simulink model "FinSimLagrange1"  (R2020b)
settings: Solver=FixedStepAuto  StartTime=0.0  StopTime=10.0  FixedStep=0.001  RelTol=1e-3
values from neighbouring files (symbols this model uses):
  m = {0 0 0 0 0}    [DynMatrixCalculator.m]    (also in DynMats_Iterative.mat = ; FinLagrange_2.m = mass{i})
  N = {zeros(3,1) zeros(3,1) zeros(3,1) zeros(3,1) zeros(3,1)}    [DynMatrixCalculator.m]    (also in DynMats_Iterative.mat = )
undefined symbols (not defined in the file or in its folder): X, Y, Z
libraries: sm_lib x34, nesl_utility x24
(part 4 of 4)

== matlab function FinSimLagrange1/Analytical Forward. Dynamics/MATLAB Function ==
  data: Tau input; theta input; theta_d input; theta_2d output; EndEffector output
function [theta_2d,EndEffector] = fcn(Tau, theta, theta_d)

q1 = theta(1);    q_d1 = theta_d(1);
q2 = theta(2);    q_d2 = theta_d(2);
q3 = theta(3);    q_d3 = theta_d(3);
q4 = theta(4);    q_d4 = theta_d(4);

%% M
M= [                                                                                                                                                                                                                                                                                                                                                                                                                                            27947/500,                                                                                                                                                                                                                                                                                                                                                                                                                                                                                                                                                                                                                                                                                                                                                                                                                                                                                                                                                                                                                                                                                                                                                                                                                                                                                                                                                                                                                                                                                                                                                                                                                                                                                                                                                                                                                                                                                                                                                                                                                                                                                                                                                                                                                                                                                                                                                                                                                                                                                                                                                                                                                                                                                                                                                                                                                                                                                                                                                                                                                                                                                                                                                                                                                                                                                                                                                                                                                                                                                                                                                                                                                                                                                                                                                                                                                                                                                                                                                                                                                                                                                                                                                                                                                                                                                                                                                                                                                                                                                                                                                                                                                                                                                                                                                                                                                                                                                                                                                                                                                                                                                                                                                                                                                                                                                                                                                                                                                                                                                                                     (252799*cos(q2))/4000000 + (8197271897754683*sin(q2))/576460752303423488 + (5271805637408845*cos(q2)*cos(q3))/36028797018963968 + (65855377368601641551*cos(q2)*sin(q3))/14073748835532800000 - (6905770129014017*cos(q2)*cos(q3)*cos(q4))/4503599627370496 + (1448762964128815*cos(q2)*cos(q3)*sin(q4))/9007199254740992 + (1448762964128815*cos(q2)*cos(q4)*sin(q3))/9007199254740992 + (6905770129014017*cos(q2)*sin(q3)*sin(q4))/4503599627370496,                                                                                                                                                                                                                                                                                                                                                                                                                                                                                                                                                                                                                                                                                                                                                                                                                                                                                                                                                                                                                                                                                                                                                                                                                                                                                                                                                                                                                                                                                                                                                                                                                                                                                                                                                                                                                                                                                                                                                                                                                                                                                                                                                                                                                                                                                                                                                                                                                                                                                                                                                                                                                                                                                                                                                                                                                                                                                                                                                                                                                                                                                                                                                                                                                                                                                                                                                                                                                               (65855377368601641551*cos(q3)*sin(q2))/14073748835532800000 - (5271805637408845*sin(q2)*sin(q3))/36028797018963968 - (1448762964128815*sin(q2)*sin(q3)*sin(q4))/9007199254740992 + (1448762964128815*cos(q3)*cos(q4)*sin(q2))/9007199254740992 + (6905770129014017*cos(q3)*sin(q2)*sin(q4))/4503599627370496 + (6905770129014017*cos(q4)*sin(q2)*sin(q3))/4503599627370496,                                                                                                                                                                                                                                                                                                                                                                                                                                                                                                                                                                                                                                                                                                                                                                                                                                                                                                                                                                                                                                                                                                                                                                                                                                                                                                                                                                                                                                                                                                                                                                                                                                                                                                                                                                                                                                                                                     (1448762964128815*cos(q3)*cos(q4)*sin(q2))/9007199254740992 - (1448762964128815*sin(q2)*sin(q3)*sin(q4))/9007199254740992 + (6905770129014017*cos(q3)*sin(q2)*sin(q4))/4503599627370496 + (6905770129014017*cos(q4)*sin(q2)*sin(q3))/4503599627370496
(252799*cos(q2))/4000000 + (8197271897754683*sin(q2))/576460752303423488 + (5271805637408845*cos(q2)*cos(q3))/36028797018963968 + (65855377368601641551*cos(q2)*sin(q3))/14073748835532800000 - (6905770129014017*cos(q2)*cos(q3)*cos(q4))/4503599627370496 + (1448762964128815*cos(q2)*cos(q3)*sin(q4))/9007199254740992 + (1448762964128815*cos(q2)*cos(q4)*sin(q3))/9007199254740992 + (6905770129014017*cos(q2)*sin(q3)*sin(q4))/4503599627370496, ((59*cos(q2))/100000 + (29*cos(q2)*sin(q3))/100)*((632657*cos(q2))/100000000 + (6181388646949611*sin(q2))/576460752303423488 + (310967*cos(q2)*sin(q3))/100000 - (6905770129014017*cos(q2)*cos(q3)*cos(q4))/4503599627370496 + (1448762964128815*cos(q2)*cos(q3)*sin(q4))/9007199254740992 + (1448762964128815*cos(q2)*cos(q4)*sin(q3))/9007199254740992 + (6905770129014017*cos(q2)*sin(q3)*sin(q4))/4503599627370496) + sin(q2)*((452416774701268201*cos(q2))/57646075230342348800000 + (315371787680421*sin(q2))/9007199254740992 - (5398328972706657*cos(q2)*cos(q3))/36893488147419103232 - (185161787713245*cos(q2)*sin(q3))/72057594037927936) + (cos(q2)*cos(q3)*cos(q4) - cos(q2)*sin(q3)*sin(q4))*((1229911296841483*sin(q2))/2305843009213693952 - (407440437611827003*cos(q2))/450359962737049600000 - (200267333741406493*cos(q2)*sin(q3))/450359962737049600 + (6760346681275207*cos(q2)*cos(q3)*cos(q4))/18014398509481984 + (8070931876976101*cos(q2)*cos(q3)*sin(q4))/576460752303423488 + (8070931876976101*cos(q2)*cos(q4)*sin(q3))/576460752303423488 - (6760346681275207*cos(q2)*sin(q3)*sin(q4))/18014398509481984) + cos(q2)*((315371787680421*cos(q2))/9007199254740992 - (452416774701268201*sin(q2))/57646075230342348800000 + (5398328972706657*cos(q3)*sin(q2))/36893488147419103232 + (185161787713245*sin(q2)*sin(q3))/72057594037927936) + (59*sin(q2)*((392409*sin(q2))/50000000 - (7668080927140139*cos(q2))/576460752303423488 + (5271805637408845*cos(q3)*sin(q2))/36028797018963968 + (7069012104707315*sin(q2)*sin(q3))/4503599627370496))/100000 + (cos(q2)*cos(q3)*sin(q4) + cos(q2)*cos(q4)*sin(q3))*((17095402976720017*cos(q2))/180143985094819840000 - (2967066550535813*sin(q2))/18446744073709551616 + (8402825191947127*cos(q2)*sin(q3))/180143985094819840 + (8070931876976101*cos(q2)*cos(q3)*cos(q4))/576460752303423488 + (23447259624965*cos(q2)*cos(q3)*sin(q4))/2251799813685248 + (23447259624965*cos(q2)*cos(q4)*sin(q3))/2251799813685248 - (8070931876976101*cos(q2)*sin(q3)*sin(q4))/576460752303423488) + sin(q2)*((364701930170027049*cos(q2))/57646075230342348800000 + (180337153490037*sin(q2))/18014398509481984 + (179260270761538719*cos(q2)*sin(q3))/57646075230342348800 + (1229911296841483*cos(q2)*cos(q3)*cos(q4))/2305843009213693952 - (2967066550535813*cos(q2)*cos(q3)*sin(q4))/18446744073709551616 - (2967066550535813*cos(q2)*cos(q4)*sin(q3))/18446744073709551616 - (1229911296841483*cos(q2)*sin(q3)*sin(q4))/2305843009213693952) + ((59*sin(q2))/100000 + (29*sin(q2)*sin(q3))/100)*((632657*sin(q2))/100000000 - (6181388646949611*cos(q2))/576460752303423488 + (310967*sin(q2)*sin(q3))/100000 + (6905770129014017*sin(q2)*sin(q3)*sin(q4))/4503599627370496 - (6905770129014017*cos(q3)*cos(q4)*sin(q2))/4503599627370496 + (1448762964128815*cos(q3)*sin(q2)*sin(q4))/9007199254740992 + (1448762964128815*cos(q4)*sin(q2)*sin(q3))/9007199254740992) + cos(q2)*((3135211865359407*cos(q2))/72057594037927936 - (3617406512854443*sin(q2))/73786976294838206464) + (sin(q2)*sin(q3)*sin(q4) - cos(q3)*cos(q4)*sin(q2))*((1229911296841483*cos(q2))/2305843009213693952 + (407440437611827003*sin(q2))/450359962737049600000 + (200267333741406493*sin(q2)*sin(q3))/450359962737049600 + (6760346681275207*sin(q2)*sin(q3)*sin(q4))/18014398509481984 - (6760346681275207*cos(q3)*cos(q4)*sin(q2))/18014398509481984 - (8070931876976101*cos(q3)*sin(q2)*sin(q4))/576460752303423488 - (8070931876976101*cos(q4)*sin(q2)*sin(q3))/576460752303423488) + (cos(q3)*sin(q2)*sin(q4) + cos(q4)*sin(q2)*sin(q3))*((2967066550535813*cos(q2))/18446744073709551616 + (17095402976720017*sin(q2))/180143985094819840000 + (8402825191947127*sin(q2)*sin(q3))/180143985094819840 - (8070931876976101*sin(q2)*sin(q3)*sin(q4))/576460752303423488 + (8070931876976101*cos(q3)*cos(q4)*sin(q2))/576460752303423488 + (23447259624965*cos(q3)*sin(q2)*sin(q4))/2251799813685248 + (23447259624965*cos(q4)*sin(q2)*sin(q3))/2251799813685248) + sin(q2)*((3617406512854443*cos(q2))/73786976294838206464 + (3135211865359407*sin(q2))/72057594037927936) + cos(q2)*((180337153490037*cos(q2))/18014398509481984 - (364701930170027049*sin(q2))/57646075230342348800000 - (179260270761538719*sin(q2)*sin(q3))/57646075230342348800 + (1229911296841483*sin(q2)*sin(q3)*sin(q4))/2305843009213693952 - (1229911296841483*cos(q3)*cos(q4)*sin(q2))/2305843009213693952 + (2967066550535813*cos(q3)*sin(q2)*sin(q4))/18446744073709551616 + (2967066550535813*cos(q4)*sin(q2)*sin(q3))/18446744073709551616) + cos(q2)*((4249992925154011*cos(q2))/288230376151711744 + (3617406512854443*sin(q2))/73786976294838206464) - sin(q2)*((3617406512854443*cos(q2))/73786976294838206464 - (4249992925154011*sin(q2))/288230376151711744) + (59*cos(q2)*((392409*cos(q2))/50000000 + (7668080927140139*sin(q2))/576460752303423488 + (5271805637408845*cos(q2)*cos(q3))/36028797018963968 + (7069012104707315*cos(q2)*sin(q3))/4503599627370496))/100000 + cos(q3)*sin(q2)*((5398328972706657*cos(q2))/36893488147419103232 + (62207306521424371*sin(q2))/720575940379279360000 + (263182111629015*cos(q3)*sin(q2))/18014398509481984 - (2055946696629407*sin(q2)*sin(q3))/144115188075855872) + cos(q2)*sin(q3)*((83414342835546317*cos(q2))/90071992547409920000 - (185161787713245*sin(q2))/72057594037927936 - (2055946696629407*cos(q2)*cos(q3))/144115188075855872 + (2929294752374665*cos(q2)*sin(q3))/9007199254740992) + sin(q2)*sin(q3)*((185161787713245*cos(q2))/72057594037927936 + (83414342835546317*sin(q2))/90071992547409920000 - (2055946696629407*cos(q3)*sin(q2))/144115188075855872 + (2929294752374665*sin(q2)*sin(q3))/9007199254740992) + cos(q2)*cos(q3)*((62207306521424371*cos(q2))/720575940379279360000 - (5398328972706657*sin(q2))/36893488147419103232 + (263182111629015*cos(q2)*cos(q3))/18014398509481984 - (2055946696629407*cos(q2)*sin(q3))/144115188075855872),                                                                                                                          cos(q2)*sin(q3)*((5398328972706657*cos(q2))/36893488147419103232 + (62207306521424371*sin(q2))/720575940379279360000 + (263182111629015*cos(q3)*sin(q2))/18014398509481984 - (2055946696629407*sin(q2)*sin(q3))/144115188075855872) - (sin(q2)*sin(q3)*sin(q4) - cos(q3)*cos(q4)*sin(q2))*((17095402976720017*cos(q2))/180143985094819840000 - (2967066550535813*sin(q2))/18446744073709551616 + (8402825191947127*cos(q2)*sin(q3))/180143985094819840 + (8070931876976101*cos(q2)*cos(q3)*cos(q4))/576460752303423488 + (23447259624965*cos(q2)*cos(q3)*sin(q4))/2251799813685248 + (23447259624965*cos(q2)*cos(q4)*sin(q3))/2251799813685248 - (8070931876976101*cos(q2)*sin(q3)*sin(q4))/576460752303423488) - (cos(q2)*cos(q3)*sin(q4) + cos(q2)*cos(q4)*sin(q3))*((1229911296841483*cos(q2))/2305843009213693952 + (407440437611827003*sin(q2))/450359962737049600000 + (200267333741406493*sin(q2)*sin(q3))/450359962737049600 + (6760346681275207*sin(q2)*sin(q3)*sin(q4))/18014398509481984 - (6760346681275207*cos(q3)*cos(q4)*sin(q2))/18014398509481984 - (8070931876976101*cos(q3)*sin(q2)*sin(q4))/576460752303423488 - (8070931876976101*cos(q4)*sin(q2)*sin(q3))/576460752303423488) - (cos(q2)*cos(q3)*cos(q4) - cos(q2)*sin(q3)*sin(q4))*((2967066550535813*cos(q2))/18446744073709551616 + (17095402976720017*sin(q2))/180143985094819840000 + (8402825191947127*sin(q2)*sin(q3))/180143985094819840 - (8070931876976101*sin(q2)*sin(q3)*sin(q4))/576460752303423488 + (8070931876976101*cos(q3)*cos(q4)*sin(q2))/576460752303423488 + (23447259624965*cos(q3)*sin(q2)*sin(q4))/2251799813685248 + (23447259624965*cos(q4)*sin(q2)*sin(q3))/2251799813685248) - sin(q2)*sin(q3)*((62207306521424371*cos(q2))/720575940379279360000 - (5398328972706657*sin(q2))/36893488147419103232 + (263182111629015*cos(q2)*cos(q3))/18014398509481984 - (2055946696629407*cos(q2)*sin(q3))/144115188075855872) - (cos(q3)*sin(q2)*sin(q4) + cos(q4)*sin(q2)*sin(q3))*((1229911296841483*sin(q2))/2305843009213693952 - (407440437611827003*cos(q2))/450359962737049600000 - (200267333741406493*cos(q2)*sin(q3))/450359962737049600 + (6760346681275207*cos(q2)*cos(q3)*cos(q4))/18014398509481984 + (8070931876976101*cos(q2)*cos(q3)*sin(q4))/576460752303423488 + (8070931876976101*cos(q2)*cos(q4)*sin(q3))/576460752303423488 - (6760346681275207*cos(q2)*sin(q3)*sin(q4))/18014398509481984) + (29*cos(q3)*sin(q2)*((632657*cos(q2))/100000000 + (6181388646949611*sin(q2))/576460752303423488 + (310967*cos(q2)*sin(q3))/100000 - (6905770129014017*cos(q2)*cos(q3)*cos(q4))/4503599627370496 + (1448762964128815*cos(q2)*cos(q3)*sin(q4))/9007199254740992 + (1448762964128815*cos(q2)*cos(q4)*sin(q3))/9007199254740992 + (6905770129014017*cos(q2)*sin(q3)*sin(q4))/4503599627370496))/100 - (29*cos(q2)*cos(q3)*((632657*sin(q2))/100000000 - (6181388646949611*cos(q2))/576460752303423488 + (310967*sin(q2)*sin(q3))/100000 + (6905770129014017*sin(q2)*sin(q3)*sin(q4))/4503599627370496 - (6905770129014017*cos(q3)*cos(q4)*sin(q2))/4503599627370496 + (1448762964128815*cos(q3)*sin(q2)*sin(q4))/9007199254740992 + (1448762964128815*cos(q4)*sin(q2)*sin(q3))/9007199254740992))/100 + cos(q3)*sin(q2)*((83414342835546317*cos(q2))/90071992547409920000 - (185161787713245*sin(q2))/72057594037927936 - (2055946696629407*cos(q2)*cos(q3))/144115188075855872 + (2929294752374665*cos(q2)*sin(q3))/9007199254740992) - cos(q2)*cos(q3)*((185161787713245*cos(q2))/72057594037927936 + (83414342835546317*sin(q2))/90071992547409920000 - (2055946696629407*cos(q3)*sin(q2))/144115188075855872 + (2929294752374665*sin(q2)*sin(q3))/9007199254740992),                                                                                                                                                                                                           - (cos(q3)*sin(q2)*sin(q4) + cos(q4)*sin(q2)*sin(q3))*((1229911296841483*sin(q2))/2305843009213693952 - (407440437611827003*cos(q2))/450359962737049600000 - (200267333741406493*cos(q2)*sin(q3))/450359962737049600 + (6760346681275207*cos(q2)*cos(q3)*cos(q4))/18014398509481984 + (8070931876976101*cos(q2)*cos(q3)*sin(q4))/576460752303423488 + (8070931876976101*cos(q2)*cos(q4)*sin(q3))/576460752303423488 - (6760346681275207*cos(q2)*sin(q3)*sin(q4))/18014398509481984) - (sin(q2)*sin(q3)*sin(q4) - cos(q3)*cos(q4)*sin(q2))*((17095402976720017*cos(q2))/180143985094819840000 - (2967066550535813*sin(q2))/18446744073709551616 + (8402825191947127*cos(q2)*sin(q3))/180143985094819840 + (8070931876976101*cos(q2)*cos(q3)*cos(q4))/576460752303423488 + (23447259624965*cos(q2)*cos(q3)*sin(q4))/2251799813685248 + (23447259624965*cos(q2)*cos(q4)*sin(q3))/2251799813685248 - (8070931876976101*cos(q2)*sin(q3)*sin(q4))/576460752303423488) - (cos(q2)*cos(q3)*sin(q4) + cos(q2)*cos(q4)*sin(q3))*((1229911296841483*cos(q2))/2305843009213693952 + (407440437611827003*sin(q2))/450359962737049600000 + (200267333741406493*sin(q2)*sin(q3))/450359962737049600 + (6760346681275207*sin(q2)*sin(q3)*sin(q4))/18014398509481984 - (6760346681275207*cos(q3)*cos(q4)*sin(q2))/18014398509481984 - (8070931876976101*cos(q3)*sin(q2)*sin(q4))/576460752303423488 - (8070931876976101*cos(q4)*sin(q2)*sin(q3))/576460752303423488) - (cos(q2)*cos(q3)*cos(q4) - cos(q2)*sin(q3)*sin(q4))*((2967066550535813*cos(q2))/18446744073709551616 + (17095402976720017*sin(q2))/180143985094819840000 + (8402825191947127*sin(q2)*sin(q3))/180143985094819840 - (8070931876976101*sin(q2)*sin(q3)*sin(q4))/576460752303423488 + (8070931876976101*cos(q3)*cos(q4)*sin(q2))/576460752303423488 + (23447259624965*cos(q3)*sin(q2)*sin(q4))/2251799813685248 + (23447259624965*cos(q4)*sin(q2)*sin(q3))/2251799813685248)
                                                                           (65855377368601641551*cos(q3)*sin(q2))/14073748835532800000 - (5271805637408845*sin(q2)*sin(q3))/36028797018963968 - (1448762964128815*sin(q2)*sin(q3)*sin(q4))/9007199254740992 + (1448762964128815*cos(q3)*cos(q4)*sin(q2))/9007199254740992 + (6905770129014017*cos(q3)*sin(q2)*sin(q4))/4503599627370496 + (6905770129014017*cos(q4)*sin(q2)*sin(q3))/4503599627370496,                                                                                                                                                                                                                                                                                                                                                                                                                                                                                                                                                                                                                                                                                                                                                                                                                                                                                                                                                                                                                                                                                                                                                                                                                                                                                                                                                                                                                                                                                                                                                                                                                                                                                                                                                                                                                                                                                                                                                                                                                         (cos(q3)*sin(q2)*sin(q4) + cos(q4)*sin(q2)*sin(q3))*((8070931876976101*cos(q2)*cos(q3)*sin(q4))/576460752303423488 - (23447259624965*cos(q2)*cos(q3)*cos(q4))/2251799813685248 - (8402825191947127*cos(q2)*cos(q3))/180143985094819840 + (8070931876976101*cos(q2)*cos(q4)*sin(q3))/576460752303423488 + (23447259624965*cos(q2)*sin(q3)*sin(q4))/2251799813685248) - sin(q2)*((2967066550535813*cos(q3)*cos(q4)*sin(q2))/18446744073709551616 - (2967066550535813*sin(q2)*sin(q3)*sin(q4))/18446744073709551616 - (179260270761538719*cos(q3)*sin(q2))/57646075230342348800 + (1229911296841483*cos(q3)*sin(q2)*sin(q4))/2305843009213693952 + (1229911296841483*cos(q4)*sin(q2)*sin(q3))/2305843009213693952) + ((59*cos(q2))/100000 + (29*cos(q2)*sin(q3))/100)*((310967*cos(q3)*sin(q2))/100000 - (1448762964128815*sin(q2)*sin(q3)*sin(q4))/9007199254740992 + (1448762964128815*cos(q3)*cos(q4)*sin(q2))/9007199254740992 + (6905770129014017*cos(q3)*sin(q2)*sin(q4))/4503599627370496 + (6905770129014017*cos(q4)*sin(q2)*sin(q3))/4503599627370496) - (cos(q2)*cos(q3)*sin(q4) + cos(q2)*cos(q4)*sin(q3))*((23447259624965*sin(q2)*sin(q3)*sin(q4))/2251799813685248 - (8402825191947127*cos(q3)*sin(q2))/180143985094819840 - (23447259624965*cos(q3)*cos(q4)*sin(q2))/2251799813685248 + (8070931876976101*cos(q3)*sin(q2)*sin(q4))/576460752303423488 + (8070931876976101*cos(q4)*sin(q2)*sin(q3))/576460752303423488) - (59*sin(q2)*((7069012104707315*cos(q2)*cos(q3))/4503599627370496 - (5271805637408845*cos(q2)*sin(q3))/36028797018963968))/100000 - (sin(q2)*sin(q3)*sin(q4) - cos(q3)*cos(q4)*sin(q2))*((200267333741406493*cos(q2)*cos(q3))/450359962737049600 - (8070931876976101*cos(q2)*cos(q3)*cos(q4))/576460752303423488 + (6760346681275207*cos(q2)*cos(q3)*sin(q4))/18014398509481984 + (6760346681275207*cos(q2)*cos(q4)*sin(q3))/18014398509481984 + (8070931876976101*cos(q2)*sin(q3)*sin(q4))/576460752303423488) + (59*cos(q2)*((7069012104707315*cos(q3)*sin(q2))/4503599627370496 - (5271805637408845*sin(q2)*sin(q3))/36028797018963968))/100000 - cos(q2)*((185161787713245*cos(q2)*cos(q3))/72057594037927936 - (5398328972706657*cos(q2)*sin(q3))/36893488147419103232) - (cos(q2)*cos(q3)*cos(q4) - cos(q2)*sin(q3)*sin(q4))*((200267333741406493*cos(q3)*sin(q2))/450359962737049600 + (8070931876976101*sin(q2)*sin(q3)*sin(q4))/576460752303423488 - (8070931876976101*cos(q3)*cos(q4)*sin(q2))/576460752303423488 + (6760346681275207*cos(q3)*sin(q2)*sin(q4))/18014398509481984 + (6760346681275207*cos(q4)*sin(q2)*sin(q3))/18014398509481984) - cos(q2)*((2967066550535813*cos(q2)*cos(q3)*cos(q4))/18446744073709551616 - (179260270761538719*cos(q2)*cos(q3))/57646075230342348800 + (1229911296841483*cos(q2)*cos(q3)*sin(q4))/2305843009213693952 + (1229911296841483*cos(q2)*cos(q4)*sin(q3))/2305843009213693952 - (2967066550535813*cos(q2)*sin(q3)*sin(q4))/18446744073709551616) - sin(q2)*((185161787713245*cos(q3)*sin(q2))/72057594037927936 - (5398328972706657*sin(q2)*sin(q3))/36893488147419103232) - ((59*sin(q2))/100000 + (29*sin(q2)*sin(q3))/100)*((310967*cos(q2)*cos(q3))/100000 + (1448762964128815*cos(q2)*cos(q3)*cos(q4))/9007199254740992 + (6905770129014017*cos(q2)*cos(q3)*sin(q4))/4503599627370496 + (6905770129014017*cos(q2)*cos(q4)*sin(q3))/4503599627370496 - (1448762964128815*cos(q2)*sin(q3)*sin(q4))/9007199254740992) - sin(q2)*sin(q3)*((2929294752374665*cos(q2)*cos(q3))/9007199254740992 + (2055946696629407*cos(q2)*sin(q3))/144115188075855872) + cos(q2)*sin(q3)*((2929294752374665*cos(q3)*sin(q2))/9007199254740992 + (2055946696629407*sin(q2)*sin(q3))/144115188075855872) + cos(q3)*sin(q2)*((2055946696629407*cos(q2)*cos(q3))/144115188075855872 + (263182111629015*cos(q2)*sin(q3))/18014398509481984) - cos(q2)*cos(q3)*((2055946696629407*cos(q3)*sin(q2))/144115188075855872 + (263182111629015*sin(q2)*sin(q3))/18014398509481984), (cos(q3)*sin(q4) + cos(q4)*sin(q3))*((8402825191947127*sin(q3))/180143985094819840 + (8070931876976101*cos(q3)*cos(q4))/576460752303423488 + (23447259624965*cos(q3)*sin(q4))/2251799813685248 + (23447259624965*cos(q4)*sin(q3))/2251799813685248 - (8070931876976101*sin(q3)*sin(q4))/576460752303423488) - sin(q3)*((2055946696629407*cos(q3))/144115188075855872 - (2929294752374665*sin(q3))/9007199254740992) + (cos(q2)*cos(q3)*sin(q4) + cos(q2)*cos(q4)*sin(q3))*((200267333741406493*cos(q2)*cos(q3))/450359962737049600 - (8070931876976101*cos(q2)*cos(q3)*cos(q4))/576460752303423488 + (6760346681275207*cos(q2)*cos(q3)*sin(q4))/18014398509481984 + (6760346681275207*cos(q2)*cos(q4)*sin(q3))/18014398509481984 + (8070931876976101*cos(q2)*sin(q3)*sin(q4))/576460752303423488) + cos(q3)*((263182111629015*cos(q3))/18014398509481984 - (2055946696629407*sin(q3))/144115188075855872) + (sin(q2)*sin(q3)*sin(q4) - cos(q3)*cos(q4)*sin(q2))*((23447259624965*sin(q2)*sin(q3)*sin(q4))/2251799813685248 - (8402825191947127*cos(q3)*sin(q2))/180143985094819840 - (23447259624965*cos(q3)*cos(q4)*sin(q2))/2251799813685248 + (8070931876976101*cos(q3)*sin(q2)*sin(q4))/576460752303423488 + (8070931876976101*cos(q4)*sin(q2)*sin(q3))/576460752303423488) + (cos(q3)*cos(q4) - sin(q3)*sin(q4))*((6760346681275207*cos(q3)*cos(q4))/18014398509481984 - (200267333741406493*sin(q3))/450359962737049600 + (8070931876976101*cos(q3)*sin(q4))/576460752303423488 + (8070931876976101*cos(q4)*sin(q3))/576460752303423488 - (6760346681275207*sin(q3)*sin(q4))/18014398509481984) + (cos(q3)*sin(q2)*sin(q4) + cos(q4)*sin(q2)*sin(q3))*((200267333741406493*cos(q3)*sin(q2))/450359962737049600 + (8070931876976101*sin(q2)*sin(q3)*sin(q4))/576460752303423488 - (8070931876976101*cos(q3)*cos(q4)*sin(q2))/576460752303423488 + (6760346681275207*cos(q3)*sin(q2)*sin(q4))/18014398509481984 + (6760346681275207*cos(q4)*sin(q2)*sin(q3))/18014398509481984) - (cos(q2)*cos(q3)*cos(q4) - cos(q2)*sin(q3)*sin(q4))*((8070931876976101*cos(q2)*cos(q3)*sin(q4))/576460752303423488 - (23447259624965*cos(q2)*cos(q3)*cos(q4))/2251799813685248 - (8402825191947127*cos(q2)*cos(q3))/180143985094819840 + (8070931876976101*cos(q2)*cos(q4)*sin(q3))/576460752303423488 + (23447259624965*cos(q2)*sin(q3)*sin(q4))/2251799813685248) + (29*sin(q3)*((310967*sin(q3))/100000 - (6905770129014017*cos(q3)*cos(q4))/4503599627370496 + (1448762964128815*cos(q3)*sin(q4))/9007199254740992 + (1448762964128815*cos(q4)*sin(q3))/9007199254740992 + (6905770129014017*sin(q3)*sin(q4))/4503599627370496))/100 + sin(q2)*sin(q3)*((2055946696629407*cos(q3)*sin(q2))/144115188075855872 + (263182111629015*sin(q2)*sin(q3))/18014398509481984) + (29*cos(q3)*sin(q2)*((310967*cos(q3)*sin(q2))/100000 - (1448762964128815*sin(q2)*sin(q3)*sin(q4))/9007199254740992 + (1448762964128815*cos(q3)*cos(q4)*sin(q2))/9007199254740992 + (6905770129014017*cos(q3)*sin(q2)*sin(q4))/4503599627370496 + (6905770129014017*cos(q4)*sin(q2)*sin(q3))/4503599627370496))/100 + cos(q2)*cos(q3)*((2929294752374665*cos(q2)*cos(q3))/9007199254740992 + (2055946696629407*cos(q2)*sin(q3))/144115188075855872) + cos(q3)*sin(q2)*((2929294752374665*cos(q3)*sin(q2))/9007199254740992 + (2055946696629407*sin(q2)*sin(q3))/144115188075855872) + (29*cos(q2)*cos(q3)*((310967*cos(q2)*cos(q3))/100000 + (1448762964128815*cos(q2)*cos(q3)*cos(q4))/9007199254740992 + (6905770129014017*cos(q2)*cos(q3)*sin(q4))/4503599627370496 + (6905770129014017*cos(q2)*cos(q4)*sin(q3))/4503599627370496 - (1448762964128815*cos(q2)*sin(q3)*sin(q4))/9007199254740992))/100 + cos(q2)*sin(q3)*((2055946696629407*cos(q2)*cos(q3))/144115188075855872 + (263182111629015*cos(q2)*sin(q3))/18014398509481984), (cos(q3)*sin(q4) + cos(q4)*sin(q3))*((8402825191947127*sin(q3))/180143985094819840 + (8070931876976101*cos(q3)*cos(q4))/576460752303423488 + (23447259624965*cos(q3)*sin(q4))/2251799813685248 + (23447259624965*cos(q4)*sin(q3))/2251799813685248 - (8070931876976101*sin(q3)*sin(q4))/576460752303423488) + (cos(q2)*cos(q3)*sin(q4) + cos(q2)*cos(q4)*sin(q3))*((200267333741406493*cos(q2)*cos(q3))/450359962737049600 - (8070931876976101*cos(q2)*cos(q3)*cos(q4))/576460752303423488 + (6760346681275207*cos(q2)*cos(q3)*sin(q4))/18014398509481984 + (6760346681275207*cos(q2)*cos(q4)*sin(q3))/18014398509481984 + (8070931876976101*cos(q2)*sin(q3)*sin(q4))/576460752303423488) + (sin(q2)*sin(q3)*sin(q4) - cos(q3)*cos(q4)*sin(q2))*((23447259624965*sin(q2)*sin(q3)*sin(q4))/2251799813685248 - (8402825191947127*cos(q3)*sin(q2))/180143985094819840 - (23447259624965*cos(q3)*cos(q4)*sin(q2))/2251799813685248 + (8070931876976101*cos(q3)*sin(q2)*sin(q4))/576460752303423488 + (8070931876976101*cos(q4)*sin(q2)*sin(q3))/576460752303423488) + (cos(q3)*cos(q4) - sin(q3)*sin(q4))*((6760346681275207*cos(q3)*cos(q4))/18014398509481984 - (200267333741406493*sin(q3))/450359962737049600 + (8070931876976101*cos(q3)*sin(q4))/576460752303423488 + (8070931876976101*cos(q4)*sin(q3))/576460752303423488 - (6760346681275207*sin(q3)*sin(q4))/18014398509481984) + (cos(q3)*sin(q2)*sin(q4) + cos(q4)*sin(q2)*sin(q3))*((200267333741406493*cos(q3)*sin(q2))/450359962737049600 + (8070931876976101*sin(q2)*sin(q3)*sin(q4))/576460752303423488 - (8070931876976101*cos(q3)*cos(q4)*sin(q2))/576460752303423488 + (6760346681275207*cos(q3)*sin(q2)*sin(q4))/18014398509481984 + (6760346681275207*cos(q4)*sin(q2)*sin(q3))/18014398509481984) - (cos(q2)*cos(q3)*cos(q4) - cos(q2)*sin(q3)*sin(q4))*((8070931876976101*cos(q2)*cos(q3)*sin(q4))/576460752303423488 - (23447259624965*cos(q2)*cos(q3)*cos(q4))/2251799813685248 - (8402825191947127*cos(q2)*cos(q3))/180143985094819840 + (8070931876976101*cos(q2)*cos(q4)*sin(q3))/576460752303423488 + (23447259624965*cos(q2)*sin(q3)*sin(q4))/2251799813685248)
                                                                                                                                                                                                (1448762964128815*cos(q3)*cos(q4)*sin(q2))/9007199254740992 - (1448762964128815*sin(q2)*sin(q3)*sin(q4))/9007199254740992 + (6905770129014017*cos(q3)*sin(q2)*sin(q4))/4503599627370496 + (6905770129014017*cos(q4)*sin(q2)*sin(q3))/4503599627370496,                                                                                                                                                                                                                                                                                                                                                                                                                                                                                                                                                                                                                                                                                                                                                                                                                                                                                                                                                                                                                                                                                                                                                                                                                                                                                                                                                                                                                                                                                                                                                                                                                                                                                                                                                                                                                                                                                                                                                                                                                                                                                                                                                                                                                                                                                                                                                                                                                                                                                                                                                                                                                                                                                                                                                                                                                                                                                                                                                                                                                                                                                                                                                                                                                                                                                                                                                                                                                                                                                                                   (cos(q3)*sin(q2)*sin(q4) + cos(q4)*sin(q2)*sin(q3))*((8070931876976101*cos(q2)*cos(q3)*sin(q4))/576460752303423488 - (23447259624965*cos(q2)*cos(q3)*cos(q4))/2251799813685248 + (8070931876976101*cos(q2)*cos(q4)*sin(q3))/576460752303423488 + (23447259624965*cos(q2)*sin(q3)*sin(q4))/2251799813685248) - (cos(q2)*cos(q3)*cos(q4) - cos(q2)*sin(q3)*sin(q4))*((8070931876976101*sin(q2)*sin(q3)*sin(q4))/576460752303423488 - (8070931876976101*cos(q3)*cos(q4)*sin(q2))/576460752303423488 + (6760346681275207*cos(q3)*sin(q2)*sin(q4))/18014398509481984 + (6760346681275207*cos(q4)*sin(q2)*sin(q3))/18014398509481984) - cos(q2)*((2967066550535813*cos(q2)*cos(q3)*cos(q4))/18446744073709551616 + (1229911296841483*cos(q2)*cos(q3)*sin(q4))/2305843009213693952 + (1229911296841483*cos(q2)*cos(q4)*sin(q3))/2305843009213693952 - (2967066550535813*cos(q2)*sin(q3)*sin(q4))/18446744073709551616) - sin(q2)*((2967066550535813*cos(q3)*cos(q4)*sin(q2))/18446744073709551616 - (2967066550535813*sin(q2)*sin(q3)*sin(q4))/18446744073709551616 + (1229911296841483*cos(q3)*sin(q2)*sin(q4))/2305843009213693952 + (1229911296841483*cos(q4)*sin(q2)*sin(q3))/2305843009213693952) - (sin(q2)*sin(q3)*sin(q4) - cos(q3)*cos(q4)*sin(q2))*((6760346681275207*cos(q2)*cos(q3)*sin(q4))/18014398509481984 - (8070931876976101*cos(q2)*cos(q3)*cos(q4))/576460752303423488 + (6760346681275207*cos(q2)*cos(q4)*sin(q3))/18014398509481984 + (8070931876976101*cos(q2)*sin(q3)*sin(q4))/576460752303423488) - ((59*sin(q2))/100000 + (29*sin(q2)*sin(q3))/100)*((1448762964128815*cos(q2)*cos(q3)*cos(q4))/9007199254740992 + (6905770129014017*cos(q2)*cos(q3)*sin(q4))/4503599627370496 + (6905770129014017*cos(q2)*cos(q4)*sin(q3))/4503599627370496 - (1448762964128815*cos(q2)*sin(q3)*sin(q4))/9007199254740992) - (cos(q2)*cos(q3)*sin(q4) + cos(q2)*cos(q4)*sin(q3))*((23447259624965*sin(q2)*sin(q3)*sin(q4))/2251799813685248 - (23447259624965*cos(q3)*cos(q4)*sin(q2))/2251799813685248 + (8070931876976101*cos(q3)*sin(q2)*sin(q4))/576460752303423488 + (8070931876976101*cos(q4)*sin(q2)*sin(q3))/576460752303423488) + ((59*cos(q2))/100000 + (29*cos(q2)*sin(q3))/100)*((1448762964128815*cos(q3)*cos(q4)*sin(q2))/9007199254740992 - (1448762964128815*sin(q2)*sin(q3)*sin(q4))/9007199254740992 + (6905770129014017*cos(q3)*sin(q2)*sin(q4))/4503599627370496 + (6905770129014017*cos(q4)*sin(q2)*sin(q3))/4503599627370496),                                                                                                                                                                                                                                                                                                                                                                                                                                                                                                                                                                                                                                                                                                                                                                                                                                                                                                                                                                                                                                                                                                                                                                                     (sin(q2)*sin(q3)*sin(q4) - cos(q3)*cos(q4)*sin(q2))*((23447259624965*sin(q2)*sin(q3)*sin(q4))/2251799813685248 - (23447259624965*cos(q3)*cos(q4)*sin(q2))/2251799813685248 + (8070931876976101*cos(q3)*sin(q2)*sin(q4))/576460752303423488 + (8070931876976101*cos(q4)*sin(q2)*sin(q3))/576460752303423488) + (cos(q3)*sin(q2)*sin(q4) + cos(q4)*sin(q2)*sin(q3))*((8070931876976101*sin(q2)*sin(q3)*sin(q4))/576460752303423488 - (8070931876976101*cos(q3)*cos(q4)*sin(q2))/576460752303423488 + (6760346681275207*cos(q3)*sin(q2)*sin(q4))/18014398509481984 + (6760346681275207*cos(q4)*sin(q2)*sin(q3))/18014398509481984) + (29*sin(q3)*((1448762964128815*cos(q3)*sin(q4))/9007199254740992 - (6905770129014017*cos(q3)*cos(q4))/4503599627370496 + (1448762964128815*cos(q4)*sin(q3))/9007199254740992 + (6905770129014017*sin(q3)*sin(q4))/4503599627370496))/100 - (cos(q2)*cos(q3)*cos(q4) - cos(q2)*sin(q3)*sin(q4))*((8070931876976101*cos(q2)*cos(q3)*sin(q4))/576460752303423488 - (23447259624965*cos(q2)*cos(q3)*cos(q4))/2251799813685248 + (8070931876976101*cos(q2)*cos(q4)*sin(q3))/576460752303423488 + (23447259624965*cos(q2)*sin(q3)*sin(q4))/2251799813685248) + (cos(q3)*sin(q4) + cos(q4)*sin(q3))*((8070931876976101*cos(q3)*cos(q4))/576460752303423488 + (23447259624965*cos(q3)*sin(q4))/2251799813685248 + (23447259624965*cos(q4)*sin(q3))/2251799813685248 - (8070931876976101*sin(q3)*sin(q4))/576460752303423488) + (cos(q2)*cos(q3)*sin(q4) + cos(q2)*cos(q4)*sin(q3))*((6760346681275207*cos(q2)*cos(q3)*sin(q4))/18014398509481984 - (8070931876976101*cos(q2)*cos(q3)*cos(q4))/576460752303423488 + (6760346681275207*cos(q2)*cos(q4)*sin(q3))/18014398509481984 + (8070931876976101*cos(q2)*sin(q3)*sin(q4))/576460752303423488) + (cos(q3)*cos(q4) - sin(q3)*sin(q4))*((6760346681275207*cos(q3)*cos(q4))/18014398509481984 + (8070931876976101*cos(q3)*sin(q4))/576460752303423488 + (8070931876976101*cos(q4)*sin(q3))/576460752303423488 - (6760346681275207*sin(q3)*sin(q4))/18014398509481984) + (29*cos(q3)*sin(q2)*((1448762964128815*cos(q3)*cos(q4)*sin(q2))/9007199254740992 - (1448762964128815*sin(q2)*sin(q3)*sin(q4))/9007199254740992 + (6905770129014017*cos(q3)*sin(q2)*sin(q4))/4503599627370496 + (6905770129014017*cos(q4)*sin(q2)*sin(q3))/4503599627370496))/100 + (29*cos(q2)*cos(q3)*((1448762964128815*cos(q2)*cos(q3)*cos(q4))/9007199254740992 + (6905770129014017*cos(q2)*cos(q3)*sin(q4))/4503599627370496 + (6905770129014017*cos(q2)*cos(q4)*sin(q3))/4503599627370496 - (1448762964128815*cos(q2)*sin(q3)*sin(q4))/9007199254740992))/100,                                                                                                                                                                                                                                                                                                                                       (sin(q2)*sin(q3)*sin(q4) - cos(q3)*cos(q4)*sin(q2))*((23447259624965*sin(q2)*sin(q3)*sin(q4))/2251799813685248 - (23447259624965*cos(q3)*cos(q4)*sin(q2))/2251799813685248 + (8070931876976101*cos(q3)*sin(q2)*sin(q4))/576460752303423488 + (8070931876976101*cos(q4)*sin(q2)*sin(q3))/576460752303423488) + (cos(q3)*sin(q2)*sin(q4) + cos(q4)*sin(q2)*sin(q3))*((8070931876976101*sin(q2)*sin(q3)*sin(q4))/576460752303423488 - (8070931876976101*cos(q3)*cos(q4)*sin(q2))/576460752303423488 + (6760346681275207*cos(q3)*sin(q2)*sin(q4))/18014398509481984 + (6760346681275207*cos(q4)*sin(q2)*sin(q3))/18014398509481984) - (cos(q2)*cos(q3)*cos(q4) - cos(q2)*sin(q3)*sin(q4))*((8070931876976101*cos(q2)*cos(q3)*sin(q4))/576460752303423488 - (23447259624965*cos(q2)*cos(q3)*cos(q4))/2251799813685248 + (8070931876976101*cos(q2)*cos(q4)*sin(q3))/576460752303423488 + (23447259624965*cos(q2)*sin(q3)*sin(q4))/2251799813685248) + (cos(q3)*sin(q4) + cos(q4)*sin(q3))*((8070931876976101*cos(q3)*cos(q4))/576460752303423488 + (23447259624965*cos(q3)*sin(q4))/2251799813685248 + (23447259624965*cos(q4)*sin(q3))/2251799813685248 - (8070931876976101*sin(q3)*sin(q4))/576460752303423488) + (cos(q2)*cos(q3)*sin(q4) + cos(q2)*cos(q4)*sin(q3))*((6760346681275207*cos(q2)*cos(q3)*sin(q4))/18014398509481984 - (8070931876976101*cos(q2)*cos(q3)*cos(q4))/576460752303423488 + (6760346681275207*cos(q2)*cos(q4)*sin(q3))/18014398509481984 + (8070931876976101*cos(q2)*sin(q3)*sin(q4))/576460752303423488) + (cos(q3)*cos(q4) - sin(q3)*sin(q4))*((6760346681275207*cos(q3)*cos(q4))/18014398509481984 + (8070931876976101*cos(q3)*sin(q4))/576460752303423488 + (8070931876976101*cos(q4)*sin(q3))/576460752303423488 - (6760346681275207*sin(q3)*sin(q4))/18014398509481984)];

%% V
V=[                                                                                                                                                                                                                                                                                                                                                                                                                                                                                                                                                                                                                                                                                                                                               0,                                                                                                                                                                                                                                                                                                                                                                                                                                                                                                                                                                                                                                                                                                                                                                                                                                                                                                                                                       (q_d4*cos(q2)*(1448762964128815*cos(q3 + q4) + 13811540258028034*sin(q3 + q4)))/9007199254740992 - q_d2*((252799*sin(q2))/4000000 - (8197271897754683*cos(q2))/576460752303423488 + (5271805637408845*cos(q3)*sin(q2))/36028797018963968 + (65855377368601641551*sin(q2)*sin(q3))/14073748835532800000 + (6905770129014017*sin(q2)*sin(q3)*sin(q4))/4503599627370496 - (6905770129014017*cos(q3)*cos(q4)*sin(q2))/4503599627370496 + (1448762964128815*cos(q3)*sin(q2)*sin(q4))/9007199254740992 + (1448762964128815*cos(q4)*sin(q2)*sin(q3))/9007199254740992) + (q_d3*cos(q2)*(18109537051610187500*cos(q3 + q4) + 172644253225350425000*sin(q3 + q4) + 526843018948813132408*cos(q3) - 16474392616902640625*sin(q3)))/112589990684262400000,                                                                                                                                                                                                                                                                                                                                                                                                                                                                                                                                                                   (q_d2*cos(q2)*(18109537051610187500*cos(q3 + q4) + 172644253225350425000*sin(q3 + q4) + 526843018948813132408*cos(q3) - 16474392616902640625*sin(q3)))/112589990684262400000 + (q_d4*sin(q2)*(13811540258028034*cos(q3 + q4) - 1448762964128815*sin(q3 + q4)))/9007199254740992 - (q_d3*sin(q2)*(18109537051610187500*sin(q3 + q4) - 172644253225350425000*cos(q3 + q4) + 16474392616902640625*cos(q3) + 526843018948813132408*sin(q3)))/112589990684262400000,                                                                                                                                                                                                                                                                                                                                     (q_d2*cos(q2)*(1448762964128815*cos(q3 + q4) + 13811540258028034*sin(q3 + q4)))/9007199254740992 + (q_d3*sin(q2)*(13811540258028034*cos(q3 + q4) - 1448762964128815*sin(q3 + q4)))/9007199254740992 + (q_d4*sin(q2)*(13811540258028034*cos(q3 + q4) - 1448762964128815*sin(q3 + q4)))/9007199254740992
(q_d4*cos(q2)*(1448762964128815*cos(q3 + q4) + 13811540258028034*sin(q3 + q4)))/18014398509481984 - (q_d2*((252799*sin(q2))/4000000 - (8197271897754683*cos(q2))/576460752303423488 + (5271805637408845*cos(q3)*sin(q2))/36028797018963968 + (65855377368601641551*sin(q2)*sin(q3))/14073748835532800000 + (6905770129014017*sin(q2)*sin(q3)*sin(q4))/4503599627370496 - (6905770129014017*cos(q3)*cos(q4)*sin(q2))/4503599627370496 + (1448762964128815*cos(q3)*sin(q2)*sin(q4))/9007199254740992 + (1448762964128815*cos(q4)*sin(q2)*sin(q3))/9007199254740992))/2 + (q_d3*cos(q2)*(18109537051610187500*cos(q3 + q4) + 172644253225350425000*sin(q3 + q4) + 526843018948813132408*cos(q3) - 16474392616902640625*sin(q3)))/225179981368524800000, (1706317924287871792479*q_d3*sin(2*q3))/1407374883553280000000 - (2055946696629407*q_d3*cos(2*q3))/72057594037927936 + (8070931876976101*q_d3*cos(2*q3 + 2*q4))/288230376151711744 + (8070931876976101*q_d4*cos(2*q3 + 2*q4))/288230376151711744 - (6572768604275487*q_d3*sin(2*q3 + 2*q4))/18014398509481984 - (6572768604275487*q_d4*sin(2*q3 + 2*q4))/18014398509481984 + (1448762964128815*q_d1*cos(q3 - q2 + q4))/36028797018963968 + (6905770129014017*q_d1*sin(q3 - q2 + q4))/18014398509481984 - (65855377368601641551*q_d1*cos(q2 + q3))/56294995342131200000 + (17095402976720017*q_d3*cos(q3 + q4))/90071992547409920000 + (17095402976720017*q_d4*cos(q3 + q4))/90071992547409920000 + (5271805637408845*q_d1*sin(q2 + q3))/144115188075855872 + (407440437611827003*q_d3*sin(q3 + q4))/225179981368524800000 + (407440437611827003*q_d4*sin(q3 + q4))/225179981368524800000 - (8197271897754683*q_d1*cos(q2))/1152921504606846976 + (3885467264747496851509*q_d3*cos(q3))/703687441776640000000000 + (200267333741406493*q_d4*cos(q4))/450359962737049600 + (252799*q_d1*sin(q2))/8000000 - (62207306521424371*q_d3*sin(q3))/360287970189639680000 - (8402825191947127*q_d4*sin(q4))/180143985094819840 + (65855377368601641551*q_d1*cos(q2 - q3))/56294995342131200000 - (200267333741406493*q_d3*cos(2*q3 + q4))/225179981368524800 - (200267333741406493*q_d4*cos(2*q3 + q4))/450359962737049600 + (5271805637408845*q_d1*sin(q2 - q3))/144115188075855872 + (8402825191947127*q_d3*sin(2*q3 + q4))/90071992547409920 + (8402825191947127*q_d4*sin(2*q3 + q4))/180143985094819840 - (1448762964128815*q_d1*cos(q2 + q3 + q4))/36028797018963968 - (6905770129014017*q_d1*sin(q2 + q3 + q4))/18014398509481984, (5398328972706657*q_d3*cos(q3))/36893488147419103232 - (31130840590942719*q_d3*sin(q3))/57646075230342348800 - (65855377368601641551*q_d1*cos(q2)*cos(q3))/28147497671065600000 - (1229911296841483*q_d3*cos(q3)*cos(q4))/2305843009213693952 - (1229911296841483*q_d4*cos(q3)*cos(q4))/2305843009213693952 + (5271805637408845*q_d1*cos(q2)*sin(q3))/72057594037927936 + (2967066550535813*q_d3*cos(q3)*sin(q4))/18446744073709551616 + (2967066550535813*q_d3*cos(q4)*sin(q3))/18446744073709551616 + (2967066550535813*q_d4*cos(q3)*sin(q4))/18446744073709551616 + (2967066550535813*q_d4*cos(q4)*sin(q3))/18446744073709551616 + (1229911296841483*q_d3*sin(q3)*sin(q4))/2305843009213693952 + (1229911296841483*q_d4*sin(q3)*sin(q4))/2305843009213693952 - (1448762964128815*q_d1*cos(q2)*cos(q3)*cos(q4))/18014398509481984 - (6905770129014017*q_d1*cos(q2)*cos(q3)*sin(q4))/9007199254740992 - (6905770129014017*q_d1*cos(q2)*cos(q4)*sin(q3))/9007199254740992 + (1448762964128815*q_d1*cos(q2)*sin(q3)*sin(q4))/18014398509481984,                                                                                                                                             (2967066550535813*q_d3*sin(q3 + q4))/18446744073709551616 - (6905770129014017*q_d1*sin(q3 - q2 + q4))/18014398509481984 - (1229911296841483*q_d3*cos(q3 + q4))/2305843009213693952 - (1229911296841483*q_d4*cos(q3 + q4))/2305843009213693952 - (1448762964128815*q_d1*cos(q3 - q2 + q4))/36028797018963968 + (2967066550535813*q_d4*sin(q3 + q4))/18446744073709551616 - (1448762964128815*q_d1*cos(q2 + q3 + q4))/36028797018963968 - (6905770129014017*q_d1*sin(q2 + q3 + q4))/18014398509481984
                                                                                                                                                                                                                                                                                    (q_d2*cos(q2)*(18109537051610187500*cos(q3 + q4) + 172644253225350425000*sin(q3 + q4) + 526843018948813132408*cos(q3) - 16474392616902640625*sin(q3)))/225179981368524800000 + (q_d4*sin(q2)*(13811540258028034*cos(q3 + q4) - 1448762964128815*sin(q3 + q4)))/18014398509481984 - (q_d3*sin(q2)*(18109537051610187500*sin(q3 + q4) - 172644253225350425000*cos(q3 + q4) + 16474392616902640625*cos(q3) + 526843018948813132408*sin(q3)))/225179981368524800000,                                                                                                                                                                                                              (2055946696629407*q_d2*cos(2*q3))/144115188075855872 - (1706317924287871792479*q_d2*sin(2*q3))/2814749767106560000000 - (8070931876976101*q_d2*cos(2*q3 + 2*q4))/576460752303423488 + (6572768604275487*q_d2*sin(2*q3 + 2*q4))/36028797018963968 - (1448762964128815*q_d1*cos(q3 - q2 + q4))/36028797018963968 - (6905770129014017*q_d1*sin(q3 - q2 + q4))/18014398509481984 - (65855377368601641551*q_d1*cos(q2 + q3))/56294995342131200000 - (17095402976720017*q_d2*cos(q3 + q4))/180143985094819840000 - (1229911296841483*q_d3*cos(q3 + q4))/4611686018427387904 - (1229911296841483*q_d4*cos(q3 + q4))/4611686018427387904 + (5271805637408845*q_d1*sin(q2 + q3))/144115188075855872 - (407440437611827003*q_d2*sin(q3 + q4))/450359962737049600000 + (2967066550535813*q_d3*sin(q3 + q4))/36893488147419103232 + (2967066550535813*q_d4*sin(q3 + q4))/36893488147419103232 - (3885467264747496851509*q_d2*cos(q3))/1407374883553280000000000 + (5398328972706657*q_d3*cos(q3))/73786976294838206464 + (62207306521424371*q_d2*sin(q3))/720575940379279360000 - (31130840590942719*q_d3*sin(q3))/115292150460684697600 - (65855377368601641551*q_d1*cos(q2 - q3))/56294995342131200000 + (200267333741406493*q_d2*cos(2*q3 + q4))/450359962737049600 - (5271805637408845*q_d1*sin(q2 - q3))/144115188075855872 - (8402825191947127*q_d2*sin(2*q3 + q4))/180143985094819840 - (1448762964128815*q_d1*cos(q2 + q3 + q4))/36028797018963968 - (6905770129014017*q_d1*sin(q2 + q3 + q4))/18014398509481984,                                                                                                                                             (200267333741406493*q_d4*cos(q4))/225179981368524800 - (5398328972706657*q_d2*cos(q3))/73786976294838206464 + (31130840590942719*q_d2*sin(q3))/115292150460684697600 - (8402825191947127*q_d4*sin(q4))/90071992547409920 + (1229911296841483*q_d2*cos(q3)*cos(q4))/4611686018427387904 + (5271805637408845*q_d1*cos(q3)*sin(q2))/72057594037927936 - (2967066550535813*q_d2*cos(q3)*sin(q4))/36893488147419103232 - (2967066550535813*q_d2*cos(q4)*sin(q3))/36893488147419103232 + (65855377368601641551*q_d1*sin(q2)*sin(q3))/28147497671065600000 - (1229911296841483*q_d2*sin(q3)*sin(q4))/4611686018427387904 - (6905770129014017*q_d1*cos(q3)*cos(q4)*sin(q2))/9007199254740992 + (1448762964128815*q_d1*cos(q3)*sin(q2)*sin(q4))/18014398509481984 + (1448762964128815*q_d1*cos(q4)*sin(q2)*sin(q3))/18014398509481984 + (6905770129014017*q_d1*sin(q2)*sin(q3)*sin(q4))/9007199254740992, (200267333741406493*q_d4*cos(q4))/450359962737049600 - (8402825191947127*q_d4*sin(q4))/180143985094819840 + (1229911296841483*q_d2*cos(q3)*cos(q4))/4611686018427387904 - (2967066550535813*q_d2*cos(q3)*sin(q4))/36893488147419103232 - (2967066550535813*q_d2*cos(q4)*sin(q3))/36893488147419103232 - (1229911296841483*q_d2*sin(q3)*sin(q4))/4611686018427387904 - (6905770129014017*q_d1*cos(q3)*cos(q4)*sin(q2))/9007199254740992 + (1448762964128815*q_d1*cos(q3)*sin(q2)*sin(q4))/18014398509481984 + (1448762964128815*q_d1*cos(q4)*sin(q2)*sin(q3))/18014398509481984 + (6905770129014017*q_d1*sin(q2)*sin(q3)*sin(q4))/9007199254740992
                                                                                                                                                                                                                                                                                                                                                                                                                                          (q_d2*cos(q2)*(1448762964128815*cos(q3 + q4) + 13811540258028034*sin(q3 + q4)))/18014398509481984 + (q_d3*sin(q2)*(13811540258028034*cos(q3 + q4) - 1448762964128815*sin(q3 + q4)))/18014398509481984 + (q_d4*sin(q2)*(13811540258028034*cos(q3 + q4) - 1448762964128815*sin(q3 + q4)))/18014398509481984,                                                                                                                                                                                                                                                                                                                                                                                                                                                                                                                                                                                                                                                                                                                 (6572768604275487*q_d2*sin(2*q3 + 2*q4))/36028797018963968 - (8070931876976101*q_d2*cos(2*q3 + 2*q4))/576460752303423488 - (1448762964128815*q_d1*cos(q3 - q2 + q4))/36028797018963968 - (6905770129014017*q_d1*sin(q3 - q2 + q4))/18014398509481984 - (17095402976720017*q_d2*cos(q3 + q4))/180143985094819840000 - (1229911296841483*q_d3*cos(q3 + q4))/4611686018427387904 - (1229911296841483*q_d4*cos(q3 + q4))/4611686018427387904 - (407440437611827003*q_d2*sin(q3 + q4))/450359962737049600000 + (2967066550535813*q_d3*sin(q3 + q4))/36893488147419103232 + (2967066550535813*q_d4*sin(q3 + q4))/36893488147419103232 - (200267333741406493*q_d2*cos(q4))/900719925474099200 + (8402825191947127*q_d2*sin(q4))/360287970189639680 + (200267333741406493*q_d2*cos(2*q3 + q4))/900719925474099200 - (8402825191947127*q_d2*sin(2*q3 + q4))/360287970189639680 - (1448762964128815*q_d1*cos(q2 + q3 + q4))/36028797018963968 - (6905770129014017*q_d1*sin(q2 + q3 + q4))/18014398509481984,                                                                                                                                                                                                                                                                             (200267333741406493*q_d4*cos(q4))/900719925474099200 - (200267333741406493*q_d3*cos(q4))/450359962737049600 + (8402825191947127*q_d3*sin(q4))/180143985094819840 - (8402825191947127*q_d4*sin(q4))/360287970189639680 + (1229911296841483*q_d2*cos(q3)*cos(q4))/4611686018427387904 - (2967066550535813*q_d2*cos(q3)*sin(q4))/36893488147419103232 - (2967066550535813*q_d2*cos(q4)*sin(q3))/36893488147419103232 - (1229911296841483*q_d2*sin(q3)*sin(q4))/4611686018427387904 - (6905770129014017*q_d1*cos(q3)*cos(q4)*sin(q2))/9007199254740992 + (1448762964128815*q_d1*cos(q3)*sin(q2)*sin(q4))/18014398509481984 + (1448762964128815*q_d1*cos(q4)*sin(q2)*sin(q3))/18014398509481984 + (6905770129014017*q_d1*sin(q2)*sin(q3)*sin(q4))/9007199254740992, (8402825191947127*q_d3*sin(q4))/360287970189639680 - (200267333741406493*q_d3*cos(q4))/900719925474099200 + (1229911296841483*q_d2*cos(q3)*cos(q4))/4611686018427387904 - (2967066550535813*q_d2*cos(q3)*sin(q4))/36893488147419103232 - (2967066550535813*q_d2*cos(q4)*sin(q3))/36893488147419103232 - (1229911296841483*q_d2*sin(q3)*sin(q4))/4611686018427387904 - (6905770129014017*q_d1*cos(q3)*cos(q4)*sin(q2))/9007199254740992 + (1448762964128815*q_d1*cos(q3)*sin(q2)*sin(q4))/18014398509481984 + (1448762964128815*q_d1*cos(q4)*sin(q2)*sin(q3))/18014398509481984 + (6905770129014017*q_d1*sin(q2)*sin(q3)*sin(q4))/9007199254740992];

%% G
G=[                                                                                                                                                                                                                                                                                                                                                    0
                                                                                                                                                                                                                                                                                                                                                    0
(6774560496562750677*cos(q3)*cos(q4))/450359962737049600 - (64604125198598210361531*sin(q3))/1407374883553280000000 - (1034328266059615389*cos(q3))/720575940379279360 - (284247293562073503*cos(q3)*sin(q4))/180143985094819840 - (284247293562073503*cos(q4)*sin(q3))/180143985094819840 - (6774560496562750677*sin(q3)*sin(q4))/450359962737049600
                                                                                                                                                                                                                             (981*192857558425360402101618243209381^(1/2)*cos(q3 + q4 + atan(1448762964128815/13811540258028034)))/900719925474099200];
 
%% T

T= [cos(q2)*cos(q3)*cos(q4) - cos(q2)*sin(q3)*sin(q4), - cos(q2)*cos(q3)*sin(q4) - cos(q2)*cos(q4)*sin(q3), sin(q2),      (1913*cos(q2)*cos(q3)*cos(q4))/5000 - (29*cos(q2)*sin(q3))/100 - (59*cos(q2))/100000 - (cos(q2)*cos(q3)*sin(q4))/50 - (cos(q2)*cos(q4)*sin(q3))/50 - (1913*cos(q2)*sin(q3)*sin(q4))/5000
                cos(q3)*sin(q4) + cos(q4)*sin(q3),                   cos(q3)*cos(q4) - sin(q3)*sin(q4),       0,                                                         (29*cos(q3))/100 + (cos(q3)*cos(q4))/50 + (1913*cos(q3)*sin(q4))/5000 + (1913*cos(q4)*sin(q3))/5000 - (sin(q3)*sin(q4))/50 + 873/2500
sin(q2)*sin(q3)*sin(q4) - cos(q3)*cos(q4)*sin(q2),   cos(q3)*sin(q2)*sin(q4) + cos(q4)*sin(q2)*sin(q3), cos(q2), q1 + (59*sin(q2))/100000 + (29*sin(q2)*sin(q3))/100 + (1913*sin(q2)*sin(q3)*sin(q4))/5000 - (1913*cos(q3)*cos(q4)*sin(q2))/5000 + (cos(q3)*sin(q2)*sin(q4))/50 + (cos(q4)*sin(q2)*sin(q3))/50
                                                0,                                                   0,       0,                                                                                                                                                                                             1];
                                            
%% end effector
EndEffector = T;

theta_2d = M\ (Tau- V*theta_d - G);
